simulink subsystem "button_to_temp_stage"  (R2024b)
settings: Solver=VariableStepAuto  StartTime=0.0  StopTime=10.0  RelTol=1e-3
settings Model: Creator=developer  LastModifiedBy=developer

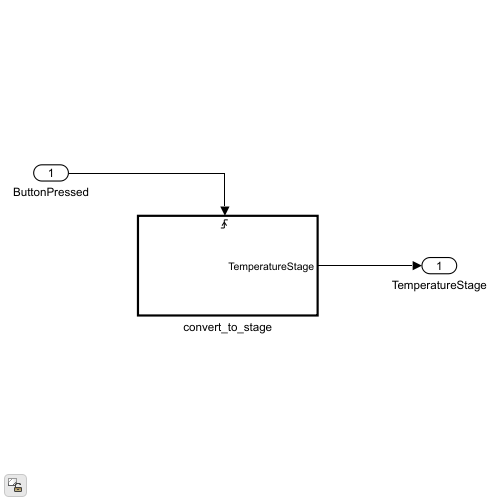
[thumbnail: Simulink's stored preview of the top-level diagram]
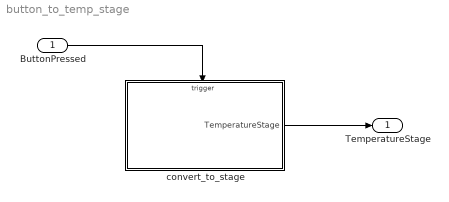
== system button_to_temp_stage ==
  ButtonPressed : Inport
  convert_to_stage : Subsystem
  TemperatureStage : Outport  OutDataTypeStr=uint8  PortDimensions=1  InitialOutput=0
  wires:
  convert_to_stage/1(TemperatureStage) -> TemperatureStage/1
  ButtonPressed/1 -> convert_to_stage/Trigger

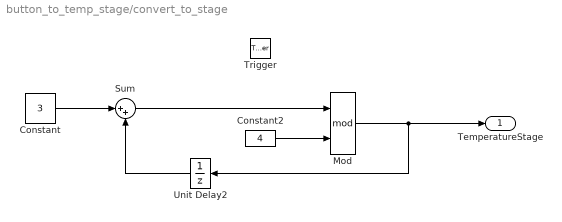
== system button_to_temp_stage/convert_to_stage ==
  Trigger : TriggerPort  VariantControl=Variant  PortDimensions=1
  Constant : Constant  Value=3  OutDataTypeStr=Inherit: Inherit via back propagation
  Constant2 : Constant  Value=4  OutDataTypeStr=Inherit: Inherit via back propagation
  Mod : Math  Operator=mod
  Sum : Sum  Inputs=|++
  Unit Delay2 : UnitDelay  SampleTime=-1  HasFrameUpgradeWarning=on
      settings: AttributesFormatString=Init = %<InitialCondition>
  TemperatureStage : Outport  InitialOutput=0
  wires:
  Unit Delay2/1 -> Sum/2
  Constant2/1 -> Mod/2
  Mod/1 -> Unit Delay2/1, TemperatureStage/1
  Constant/1 -> Sum/1
  Sum/1 -> Mod/1
